simulink model "PI_Controller_ref"  (R2020b)
settings: Solver=ode45  StartTime=0.0  StopTime=10  RelTol=1e-3
values from neighbouring files (symbols this model uses):
  Ki = 40.0    [Dictionary.sldd]
  Kp = 800.0    [Dictionary.sldd]
settings Model: DataDictionary=Dictionary.sldd  Creator=abhin  LastModifiedBy=abhin
settings DataIOCC: SaveOutput=off  SaveTime=off

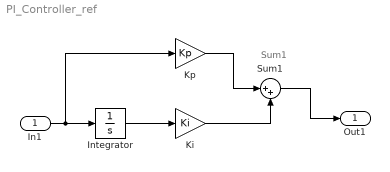
== system PI_Controller_ref ==
  note: Sum1
  In1 : Inport  OutDataTypeStr=double  PortDimensions=1  SampleTime=0
  Integrator : Integrator
  Ki : Gain  Gain=Ki
  Kp : Gain  Gain=Kp
  Sum1 : Sum  Inputs=|++
  Out1 : Outport  OutDataTypeStr=double  PortDimensions=1  SampleTime=0
  wires:
  Ki/1 -> Sum1/2
  Kp/1 -> Sum1/1
  Sum1/1 -> Out1/1
  Integrator/1 -> Ki/1
  In1/1 -> Integrator/1, Kp/1
